simulink model "GSFR_without_feedback"  (R2019b)
settings: Solver=VariableStepAuto  StartTime=0  StopTime=20.0  MaxStep=0.01  RelTol=1e-3
model workspace (MAT data in the model file):
  H = [8 1]
settings Model: EnablePacing=on  PacingRate=1000  ParameterArgumentNames=H  OrderedModelArguments=off  Creator=ruiva  LastModifiedBy=ruiva

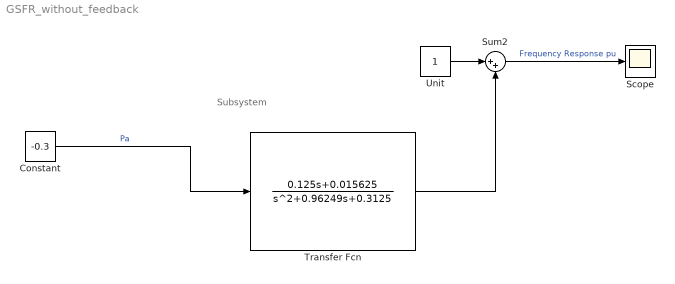
== system GSFR_without_feedback ==
  note: Subsystem
  Constant : Constant  Value=-0.3
  Scope : Scope
  Sum2 : Sum  Inputs=|++
  Transfer Fcn : TransferFcn  Numerator=[0.125 0.015625]  Denominator=[1 0.96249 0.3125]
  Unit : Constant
  wires:
  Transfer Fcn/1 -> Sum2/2
  Unit/1 -> Sum2/1
  Sum2/1 -> Scope/1  "Frequency Response pu"
  Constant/1 -> Transfer Fcn/1  "Pa"
